simulink model "apilot3"  (Simulink 2.09)
settings: Solver=ode45  StartTime=0.0  StopTime=45  MaxStep=0.033  RelTol=1e-07  AbsTol=1e-05
values from neighbouring files (symbols this model uses):
  CD = 0    [apinit.m]    (also in vorinit.m)
  gamgs = -3*pi/180    (= -0.0523598775598)    [apinit.m]    (also in ilsinit.m = -3)
  HRW = 0    [apinit.m]    (also in ilsinit.m)
  Sgs = 625/abs(gamgs)    [apinit.m]    (also in ilsinit.m)
  Sloc = 1.4*xloc    (= 2800)    [apinit.m]    (also in ilsinit.m)
  xgs = 300    [apinit.m]    (also in ilsinit.m)
  xloc = 2000    [apinit.m]    (also in ilsinit.m)
  ymod1A = [1 1 1 0 0]'    [apmode.m]
  ymod1S = [1 1 1 0 0]'    [apmode.m]
  ymod2A = [1 1 0 0 1]'    [apmode.m]
  ymod2S = [1 1 0 0 1]'    [apmode.m]
  yrefA = [0 Dpsir]'    [apmode.m]
  yrefS = [0 0 DHdotr]'    [apmode.m]
undefined symbols (not defined in the file or in its folder): Aail, Aelv, AM, Arud, Bail, Belv, Brud, Cail, Celv, Crud, Dail, Delv, Drud, GM1, sfunyst, uaero0, uprop0, xdot0, xfix, xinco
libraries: navlib1 x5, wndlib2 x3, navlib2 x2, wndlib1 x1
(part 1 of 2)
settings Model: SaveTime=off  SaveOutput=off  ConsistencyChecking=off  RTWTemplateMakefile=grt_vc.tmf

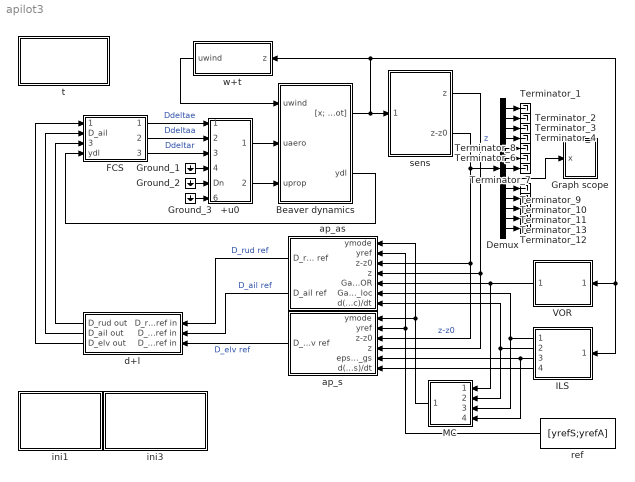
== system apilot3 ==
  +u0 : Subsystem
      mask Display: disp('Add\ninitial\ninputs')
  Beaver dynamics : Subsystem
  Demux : Demux  Outputs=13
  FCS : Subsystem
      mask Display: disp('Actuator &\ncable dy-\nnamics')
  Graph scope : Subsystem  mask(Storage scope.){npts=100, color='g-'}
      mask prompts: npts "Initial Time Range:"; color "Initial y-min:"
      mask help:
      | Storage scope using MATLAB graph window.
      | Enter plotting ranges and line type.
      mask init:
      | close all; ax = [0, @1, @2, @3];
      mask Help: Uses MATLAB's graph window.\nUse only one block per system.\nLine type must be in quotes.\nSee the M-file sfunyst.m.
      mask Display: plot(0,0,100,100,[83,76,63,52,42,38,28,16,11,84,11,11,11,90,90,11],[75,58,47,54,72,80,84,74,65,65,65,90,40,40,90,90])
  Ground_1 : Ground
  Ground_2 : Ground
  Ground_3 : Ground
  ILS : Subsystem  Orientation=left
      mask Display: plot(0,0,100,100,[53,23,30,61,53],[45,60,64,49,45],[16,27,32,26],[48,40,43,47],[21,20,24,26,21],[44,55,56,47,44],[20,20,16],[50,50,48],[38,27,26,33],[52,46,48,55],[42,38,27],[50,47,46],[40,44,44,45,45,44,42],[48,44,42,42,44,44,50],[47,45,43],[55,58,58],[54,84,98,90,54],[36,21,56,58,36],[74,68],[34,29],[81,76],[43,38],[87,83],[49,45],[94,89],[57,52],[105,105],[0,0])
  MC : Subsystem  Orientation=left
      mask Display: disp('Mode\nCon-\ntroller')
  Terminator_{1..4,6..13} (12 alike) : Terminator
  VOR : Subsystem  Orientation=left
      mask Display: plot(0,0,100,100,[86,85,90,86,80,85,0],[16,80,20,16,20,80,62],[22,18,25,28,22,19],[36,32,29,33,36,45],[17,15,12,18,16,19],[37,37,34,32,44,46],[22,31,47,52,19,15,28,22],[36,44,39,44,55,50,45,38],[31,28],[44,45],[20,18,17],[31,30,32],[36,35,36,37,36,35,35,35,33,31,25],[41,38,33,32,30,30,32,33,37,35,34],[85,42],[80,50],[86,87,87,86,84,83,84,85],[83,81,78,76,76,79,82,83])
  ap_as : Subsystem  Orientation=left
      mask Display: disp('Asymmetrical\nautopilot\nmodes')
  ap_s : Subsystem  Orientation=left
      mask Display: disp('Symmetrical\nautopilot\nmodes')
  d+l : Subsystem  Orientation=left
      mask Display: disp('computational\ndelay & limiters')
  ini1 : Subsystem
      settings: OpenFcn=apinit
      mask Type: apinit
      mask Display: disp('1. Initialize\nsubsystems\n\nAPINIT')
  ini3 : Subsystem
      settings: OpenFcn=apmode
      mask Type: apmode
      mask Display: disp('2. Select mode &\nreference signals\n\nAPMODE')
  ref : Constant  Orientation=left  Value=[yrefS;yrefA]
      mask Display: disp('Reference\nsignals')
  sens : Subsystem
      mask Display: disp('Sensors\n\nsubtract\ninitial\nconditions')
  t : Subsystem
      settings: OpenFcn=fdchelp apilot
      mask Display: disp('Apilot3\nMarc Rauw\nJune 2000')
  w+t : Subsystem  Orientation=left
      mask Display: disp('wind &\nturbulence')
  wires:
  Demux/8 -> Graph scope/1(x)
  Demux/5 -> Terminator_8/1
  Demux/6 -> Terminator_6/1
  Demux/13 -> Terminator_12/1
  Demux/12 -> Terminator_13/1
  Demux/11 -> Terminator_11/1
  Demux/10 -> Terminator_10/1
  Demux/9 -> Terminator_9/1
  Demux/4 -> Terminator_4/1
  Demux/7 -> Terminator_7/1
  Demux/3 -> Terminator_3/1
  Demux/2 -> Terminator_2/1
  Demux/1 -> Terminator_1/1
  Ground_3/1 -> +u0/6(Dpz)
  Ground_2/1 -> +u0/5(Dn)
  Ground_1/1 -> +u0/4(Ddeltaf)
  Beaver dynamics/1("[x; Hdot]") -> ILS/1("[x' ; Hdot]'"), VOR/1("[x' ; Hdot]'"), w+t/1(z), sens/1("[x; Hdot]")
  Beaver dynamics/2(ydl) -> FCS/4(ydl)
  VOR/1(Gamma_VOR) -> MC/1(Gamma_VOR), ap_as/5(Gamma_VOR)
  ap_s/1(D_elv ref) -> d+l/3(D_elv ref in)  "D_elv ref"
  d+l/3(D_elv out) -> FCS/1(D_elv)
  d+l/2(D_ail out) -> FCS/2(D_ail)
  d+l/1(D_rud out) -> FCS/3(D_rud)
  ref/1 -> ap_s/2(yref), ap_as/2(yref)
  MC/1(ymode) -> ap_s/1(ymode), ap_as/1(ymode)
  +u0/1(uaero) -> Beaver dynamics/2(uaero)
  sens/1(z) -> ap_as/4(z), ap_s/4(z)  "z"
  +u0/2(uprop) -> Beaver dynamics/3(uprop)
  FCS/1(Ddeltae) -> +u0/1(Ddeltae)  "Ddeltae"
  FCS/2(Ddeltaa) -> +u0/2(Ddeltaa)  "Ddeltaa"
  FCS/3(Ddeltar) -> +u0/3(Ddeltar)  "Ddeltar"
  ap_as/1(D_rud ref) -> d+l/1(D_rud ref in)  "D_rud ref"
  ap_as/2(D_ail ref) -> d+l/2(D_ail ref in)  "D_ail ref"
  w+t/1(uwind) -> Beaver dynamics/1(uwind)
  sens/2(z-z0) -> ap_s/3(z-z0), ap_as/3(z-z0), Demux/1  "z-z0"
  ILS/1(Gamma_loc) -> MC/3(Gamma_loc), ap_as/6(Gamma_loc)
  ILS/2(d(Gamma_loc)/dt) -> ap_as/7(d(Gamma_loc)/dt), MC/2(d(Gamma_loc)/dt)
  ILS/4(d(epsilon_gs)/dt) -> ap_s/6(d(epsilon_gs)/dt)
  ILS/3(epsilon_gs) -> ap_s/5(epsilon_gs), MC/4(epsilon_gs)

== system apilot3/+u0 ==
  note: AERODYNAMIC INPUTS:
  note: ENGINE INPUTS:
  note: Add initial inputs
  Ddeltae : Inport  Port=1  PortWidth=-1  SampleTime=-1
  Ddeltaa : Inport  Port=2  PortWidth=-1  SampleTime=-1
  Ddeltar : Inport  Port=3  PortWidth=-1  SampleTime=-1
  Ddeltaf : Inport  Port=4  PortWidth=-1  SampleTime=-1
  Dn : Inport  Port=5  PortWidth=-1  SampleTime=-1
  Dpz : Inport  Port=6  PortWidth=-1  SampleTime=-1
  Initial inputs for aeromod : Constant  Value=uaero0
  Initial inputs for engmod : Constant  Value=uprop0
  Mux1 : Mux  Inputs=4
  Mux2 : Mux  Inputs=2
  Sum : Sum  Inputs=++
  Sum1 : Sum  Inputs=++
  uaero : Outport  Port=1  InitialOutput=0
  uprop : Outport  Port=2  InitialOutput=0
  wires:
  Mux1/1 -> Sum1/2
  Sum1/1 -> uaero/1
  Initial inputs for aeromod/1 -> Sum1/1
  Ddeltaf/1 -> Mux1/4
  Ddeltar/1 -> Mux1/3
  Ddeltae/1 -> Mux1/1
  Ddeltaa/1 -> Mux1/2
  Sum/1 -> uprop/1
  Mux2/1 -> Sum/1
  Initial inputs for engmod/1 -> Sum/2
  Dn/1 -> Mux2/1
  Dpz/1 -> Mux2/2

== system apilot3/Beaver dynamics ==
  note: Beaver dynamics
      | and output equations
  uwind : Inport  Port=1  PortWidth=6  SampleTime=-1
  uaero : Inport  Port=2  PortWidth=4  SampleTime=-1
  uprop : Inport  Port=3  PortWidth=2  SampleTime=-1
  0 : Subsystem
      settings: OpenFcn=fdchelp level1
      mask Display: disp('Subsystem equivalent of\nthe S-function BEAVER\nM.O. Rauw, October 1997')
  AC : Subsystem
  Clock : Clock
  Demux1 : Demux  Outputs=[11 1]
  Mux : Mux  Inputs=[12 1]
  Mux_in : Mux  Orientation=up  Inputs=[4 2 6]
      settings: OpenFcn=fdchelp inputs
      mask Display: disp('Mux\nclick\n2x for\ninfo!')
  Mux_out : Mux  Orientation=up  Inputs=[12 12 3 3 3 4 2 6 6 6 6 6 3 3 5 3 3 3]
      settings: OpenFcn=fdchelp outputs
      mask Display: disp('Mux\n\nDouble-click for info!')
  Terminator_1 : Terminator
  To Workspace : ToWorkspace  VariableName=Out  SampleTime=0
      settings: Orientation=up  Buffer=5000
  "To Workspace " : ToWorkspace  VariableName=In  SampleTime=0
      settings: Orientation=up  Buffer=5000
  "To Workspace  " : ToWorkspace  VariableName=time  SampleTime=0
      settings: Buffer=5000
  "[x; Hdot]" : Outport  Port=1  InitialOutput=0
  ydl : Outport  Port=2  InitialOutput=0
  wires:
  AC/7(ypow) -> Mux_out/7
  Mux_in/1 -> "To Workspace "/1
  Mux_out/1 -> To Workspace/1
  Clock/1 -> "To Workspace  "/1
  AC/2(xdot) -> Mux_out/2, Demux1/1  "xdot"
  AC/15(yatm) -> Mux_out/15
  AC/14(Fwind) -> Mux_out/14
  AC/13(Fgrav) -> Mux_out/13
  AC/12(FMprop) -> Mux_out/12
  AC/11(FMaero) -> Mux_out/11
  AC/10(Cprop) -> Mux_out/10
  AC/9(Caero) -> Mux_out/9
  AC/8(yacc) -> Mux_out/8
  AC/6(yfp) -> Mux_out/6
  AC/5(ydl) -> ydl/1, Mux_out/5
  AC/16(yad1) -> Mux_out/16
  AC/3(ybvel) -> Mux_out/3
  AC/1(x) -> Mux/1, Mux_out/1  "x"
  AC/4(yuvw) -> Mux_out/4
  AC/17(yad2) -> Mux_out/17
  AC/18(yad3) -> Mux_out/18
  uwind/1 -> AC/3(" uwind"), Mux_in/3
  uprop/1 -> AC/2(uprop), Mux_in/2
  uaero/1 -> AC/1(uaero), Mux_in/1
  Demux1/1 -> Terminator_1/1
  Demux1/2 -> Mux/2  "Hdot"
  Mux/1 -> "[x; Hdot]"/1

== system apilot3/FCS ==
  note: Actuators
      | + cables:
  D_elv : Inport  Port=1  PortWidth=-1  SampleTime=-1
  D_ail : Inport  Port=2  PortWidth=-1  SampleTime=-1
  D_rud : Inport  Port=3  PortWidth=-1  SampleTime=-1
  ydl : Inport  Port=4  PortWidth=-1  SampleTime=-1
  Demux1 : Demux  Outputs=3
  Mux1 : Mux  Inputs=2
  Mux2 : Mux  Inputs=2
  Mux3 : Mux  Inputs=2
  ailerons : StateSpace  A=Aail  B=Bail  C=Cail*2  D=Dail  X0=0
  elevator : StateSpace  A=Aelv  B=Belv  C=Celv  D=Delv  X0=0
  rudder : StateSpace  A=Arud  B=Brud  C=Crud  D=Drud  X0=0
  t : Subsystem
      settings: OpenFcn=fdchelp actuatr
      mask Display: disp('Actuator & cable dynamics\nMarc Rauw, October 1997')
  Ddeltae : Outport  Port=1  InitialOutput=0
  Ddeltaa : Outport  Port=2  InitialOutput=0
  Ddeltar : Outport  Port=3  InitialOutput=0
  wires:
  D_rud/1 -> Mux3/1
  D_ail/1 -> Mux2/1
  D_elv/1 -> Mux1/1
  rudder/1 -> Ddeltar/1
  ydl/1 -> Demux1/1
  ailerons/1 -> Ddeltaa/1
  elevator/1 -> Ddeltae/1
  Mux3/1 -> rudder/1
  Mux2/1 -> ailerons/1
  Mux1/1 -> elevator/1
  Demux1/3 -> Mux3/2
  Demux1/1 -> Mux2/2
  Demux1/2 -> Mux1/2

== system apilot3/Graph scope ==
  x : Inport  Port=1  PortWidth=-1  SampleTime=-1
  "S-function M-file which plots lines " : S-Function  LoadFcn=sfunyst([],[],[],'LoadBlock')  FunctionName=sfunyst  Parameters=ax, color, npts
      settings: CopyFcn=sfunyst([],[],[],'CopyBlock')  DeleteFcn=sfunyst([],[],[],'DeleteBlock')
  wires:
  x/1 -> "S-function M-file which plots lines "/1

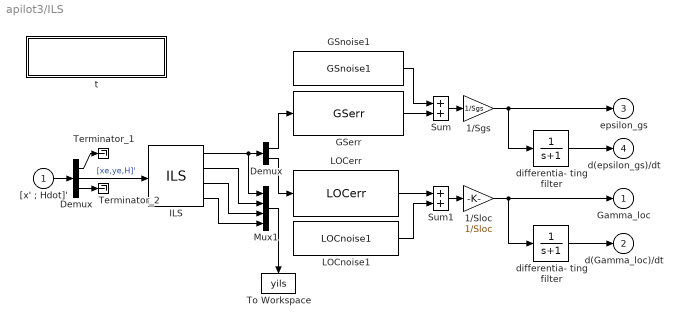
== system apilot3/ILS ==
  "[x' ; Hdot]'" : Inport  Port=1  PortWidth=-1  SampleTime=-1
  1/Sgs : Gain  Gain=1/Sgs
  1/Sloc : Gain  Gain=1/Sloc
  Demux : Demux  Outputs=2
  "Demux " : Demux  Outputs=[9 3 1]
  GSerr : navlib1/GSerr  cat=2  MaskParam2=100  MaskParam3=100  MaskParam4=-3
  GSnoise1 : navlib1/GSnoise1  Lgs=85  sigma_gs=15  V=40
  ILS : navlib1/ILS  RWpos=[20000,-100,0]  MaskParam1=0  MaskParam3=2200  MaskParam4=300  MaskParam5=100  MaskParam6=3
  LOCerr : navlib1/LOCerr  cat=2  xloc=2200  MaskParam2=100  MaskParam3=100
  LOCnoise1 : navlib1/LOCnoise1  Lloc=130  sigma_loc=15  V=40
  Mux1 : Mux  Inputs=[2 2 6 2]
  Sum : Sum  Inputs=++
  Sum1 : Sum  Inputs=++
  Terminator_1 : Terminator
  Terminator_2 : Terminator
  To Workspace : ToWorkspace  VariableName=yils  SampleTime=0
      settings: Orientation=down  Buffer=5000
  differentia- ting filter : TransferFcn  Numerator=[1]  Denominator=[1 1]
  "differentia- ting filter " : TransferFcn  Numerator=[1]  Denominator=[1 1]
  t : Subsystem
      mask Display: disp('ILS signals\nMarc Rauw, January 1998')
  Gamma_loc : Outport  Port=1  InitialOutput=0
  d(Gamma_loc)/dt : Outport  Port=2  InitialOutput=0
  epsilon_gs : Outport  Port=3  InitialOutput=0
  d(epsilon_gs)/dt : Outport  Port=4  InitialOutput=0
  wires:
  1/Sgs/1 -> epsilon_gs/1, "differentia- ting filter "/1
  "differentia- ting filter "/1 -> d(epsilon_gs)/dt/1
  1/Sloc/1 -> Gamma_loc/1, differentia- ting filter/1
  differentia- ting filter/1 -> d(Gamma_loc)/dt/1
  Mux1/1 -> To Workspace/1
  Demux/1 -> GSerr/1
  Demux/2 -> LOCerr/1
  GSerr/1 -> Sum/2
  LOCnoise1/1 -> Sum1/2
  Sum/1 -> 1/Sgs/1
  Sum1/1 -> 1/Sloc/1
  ILS/4 -> Mux1/4
  ILS/1 -> Demux/1, Mux1/1
  ILS/3 -> Mux1/3
  GSnoise1/1 -> Sum/1
  ILS/2 -> Mux1/2
  LOCerr/1 -> Sum1/1
  "Demux "/3 -> Terminator_2/1
  "Demux "/1 -> Terminator_1/1
  "Demux "/2 -> ILS/1  "[xe,ye,H]'"
  "[x' ; Hdot]'"/1 -> "Demux "/1

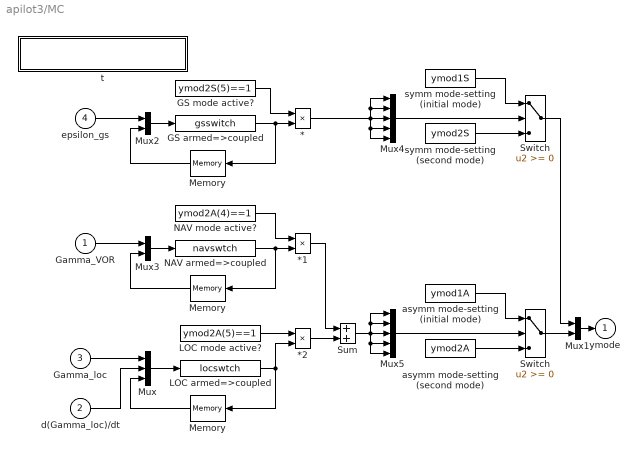
== system apilot3/MC ==
  Gamma_VOR : Inport  Port=1  PortWidth=-1  SampleTime=-1
  d(Gamma_loc)/dt : Inport  Port=2  PortWidth=-1  SampleTime=-1
  Gamma_loc : Inport  Port=3  PortWidth=-1  SampleTime=-1
  epsilon_gs : Inport  Port=4  PortWidth=-1  SampleTime=-1
  " Memory" : Memory  Orientation=left  X0=0  InheritSampleTime=off
  * : Product  Inputs=2
  *1 : Product  Inputs=2
  *2 : Product  Inputs=2
  GS armed=>coupled : MATLABFcn  MATLABFcn=gsswitch  OutputWidth=1
      mask Display: disp('gsswitch.m')
  GS mode active? : Constant  Value=ymod2S(5)==1
  LOC armed=>coupled : MATLABFcn  MATLABFcn=locswtch  OutputWidth=1
      mask Display: disp('locswtch.m')
  LOC mode active? : Constant  Value=ymod2A(5)==1
  Memory : Memory  Orientation=left  X0=1  InheritSampleTime=off
  "Memory " : Memory  Orientation=left  X0=0  InheritSampleTime=off
  Mux : Mux  Inputs=3
  Mux1 : Mux  Inputs=[5 5]
  Mux2 : Mux  Inputs=2
  Mux3 : Mux  Inputs=2
  Mux4 : Mux  Inputs=5
  Mux5 : Mux  Inputs=5
  NAV armed=>coupled : MATLABFcn  MATLABFcn=navswtch  OutputWidth=1
      mask Display: disp('navswtch.m')
  NAV mode active? : Constant  Value=ymod2A(4)==1
  Sum : Sum  Inputs=++
  Switch : Switch  Threshold=0
  "Switch " : Switch  Threshold=0
  asymm mode-setting (initial mode) : Constant  Value=ymod1A
  asymm mode-setting (second mode) : Constant  Value=ymod2A
  symm mode-setting (initial mode) : Constant  Value=ymod1S
  symm mode-setting (second mode) : Constant  Value=ymod2S
  t : Subsystem
      settings: OpenFcn=fdchelp modectrl
      mask Display: disp('Mode-controller\nM.O. Rauw, October 1997')
  ymode : Outport  Port=1  InitialOutput=0
  wires:
  asymm mode-setting (initial mode)/1 -> "Switch "/1
  symm mode-setting (initial mode)/1 -> Switch/1
  *1/1 -> Sum/1
  Sum/1 -> Mux5/2, Mux5/1, Mux5/4, Mux5/5, Mux5/3
  Switch/1 -> Mux1/1
  symm mode-setting (second mode)/1 -> Switch/3
  " Memory"/1 -> Mux/3
  "Memory "/1 -> Mux3/2
  Memory/1 -> Mux2/2
  */1 -> Mux4/4, Mux4/5, Mux4/2, Mux4/1, Mux4/3
  LOC armed=>coupled/1 -> " Memory"/1, *2/2
  asymm mode-setting (second mode)/1 -> "Switch "/3
  *2/1 -> Sum/2
  LOC mode active?/1 -> *2/1
  NAV mode active?/1 -> *1/1
  NAV armed=>coupled/1 -> *1/2, "Memory "/1
  GS mode active?/1 -> */1
  Mux1/1 -> ymode/1
  "Switch "/1 -> Mux1/2
  GS armed=>coupled/1 -> */2, Memory/1
  Mux5/1 -> "Switch "/2
  Mux4/1 -> Switch/2
  d(Gamma_loc)/dt/1 -> Mux/2
  Gamma_VOR/1 -> Mux3/1
  Mux3/1 -> NAV armed=>coupled/1
  epsilon_gs/1 -> Mux2/1
  Mux2/1 -> GS armed=>coupled/1
  Gamma_loc/1 -> Mux/1
  Mux/1 -> LOC armed=>coupled/1

== system apilot3/VOR ==
  "[x' ; Hdot]'" : Inport  Port=1  PortWidth=-1  SampleTime=-1
  Demux : Demux  Outputs=[6 1 2 3 1]
  Mux1 : Mux  Inputs=[1 1 2 1]
  Terminator_1 : Terminator
  Terminator_2 : Terminator
  Terminator_3 : Terminator
  To Workspace : ToWorkspace  VariableName=yvor  SampleTime=0
      settings: Buffer=5000
  VOR : navlib2/VOR  xVOR=xVOR  yVOR=yVOR  HVOR=HVOR  MaskParam4=CD
  VORERR : navlib2/VORERR  MaskParam1=5
  t : Subsystem
      mask Display: disp('VOR signals\nMarc Rauw, January 1998')
  Gamma_VOR : Outport  Port=1  InitialOutput=0
  wires:
  VOR/1 -> VORERR/1
  Mux1/1 -> To Workspace/1
  VOR/2 -> Mux1/2
  VOR/3 -> Mux1/3
  VOR/4 -> Mux1/4
  VORERR/1 -> Gamma_VOR/1, Mux1/1
  "[x' ; Hdot]'"/1 -> Demux/1
  Demux/5 -> Terminator_3/1
  Demux/3 -> Terminator_2/1
  Demux/1 -> Terminator_1/1
  Demux/4 -> VOR/1  "[xe,ye,H]'"
  Demux/2 -> VOR/2  "psi"

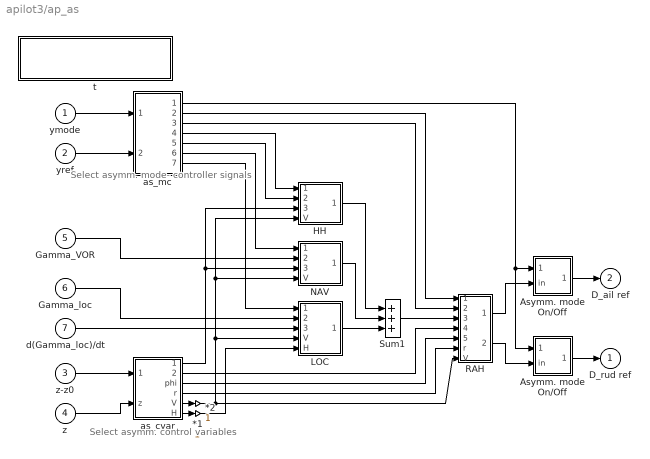
== system apilot3/ap_as ==
  note: Select asymm.
      | control variables
  note: Select asymm. mode-
      | controller signals
  ymode : Inport  Port=1  PortWidth=-1  SampleTime=-1
  yref : Inport  Port=2  PortWidth=-1  SampleTime=-1
  z-z0 : Inport  Port=3  PortWidth=-1  SampleTime=-1
  z : Inport  Port=4  PortWidth=-1  SampleTime=-1
  Gamma_VOR : Inport  Port=5  PortWidth=-1  SampleTime=-1
  Gamma_loc : Inport  Port=6  PortWidth=-1  SampleTime=-1
  d(Gamma_loc)/dt : Inport  Port=7  PortWidth=-1  SampleTime=-1
  *1 : Gain  Gain=1
  *2 : Gain  Gain=1
  Asymm. mode On/Off : Subsystem
      mask Type: On/off switch
      mask Description:
      | If input(1) = 1
      |      output = input(2)
      |  else if input(1) = 0
      |      output = 0
      mask Help: On/off switch.
      mask Display: plot(0,0,100,100,[31,31,32,34,34,32,31,31,0],[50,48,47,48,51,53,51,50,50],[100,75,51],[50,50,97]);disp('?')
  "Asymm. mode On/Off " : Subsystem
      mask Type: On/off switch
      mask Description:
      | If input(1) = 1
      |      output = input(2)
      |  else if input(1) = 0
      |      output = 0
      mask Help: On/off switch.
      mask Display: plot(0,0,100,100,[31,31,32,34,34,32,31,31,0],[50,48,47,48,51,53,51,50,50],[100,75,51],[50,50,97]);disp('?')
  HH : Subsystem
  LOC : Subsystem
  NAV : Subsystem
  RAH : Subsystem
  Sum1 : Sum  Inputs=+++
  as_cvar : Subsystem
  as_mc : Subsystem
  t : Subsystem
      settings: OpenFcn=fdchelp ap_asymm
      mask Display: disp('Asymm. autopilot modes\nMarc Rauw, October 1997')
  D_rud ref : Outport  Port=1  InitialOutput=0
  D_ail ref : Outport  Port=2  InitialOutput=0
  wires:
  as_mc/1(asymm. mode?) -> Asymm. mode On/Off/1(crit), "Asymm. mode On/Off "/1(crit)
  HH/1(Dphir (HH)) -> Sum1/1
  RAH/2(D_rud ref) -> Asymm. mode On/Off/2(in)
  RAH/1(D_ail ref) -> "Asymm. mode On/Off "/2(in)
  as_cvar/1(psi-psi0) -> NAV/3(psi-psi0), HH/3(psi-psi0)
  z-z0/1 -> as_cvar/1(z-z0)
  Asymm. mode On/Off/1(out) -> D_rud ref/1
  "Asymm. mode On/Off "/1(out) -> D_ail ref/1
  yref/1 -> as_mc/2(yref)
  ymode/1 -> as_mc/1(ymode)
  NAV/1(Dphir (NAV)) -> Sum1/2
  LOC/1(Dphir (LOC)) -> Sum1/3
  as_cvar/5(V) -> *1/1
  as_cvar/4(r) -> RAH/6(r)
  as_cvar/3(phi) -> RAH/5(phi)
  as_cvar/2(phi-phi0) -> RAH/4(phi-phi0)
  as_mc/2(asymm. out. loop?) -> RAH/1(Asymm out. loop?)
  as_mc/3(Dphir (RAH)) -> RAH/2(Dphir (RAH))
  as_mc/4(HH?) -> HH/1(HH?)
  as_mc/6(NAV?) -> NAV/1(NAV?)
  as_mc/7(LOC coupled?) -> LOC/1(LOC coupled?)
  as_cvar/6(H) -> *2/1
  *1/1 -> NAV/4(V), HH/4(V), LOC/4(V), RAH/7(V)
  *2/1 -> LOC/5(H)
  Sum1/1 -> RAH/3(Dphir (out. loop))
  as_mc/5(Dpsir (HH)) -> HH/2(Dpsir (HH))
  Gamma_VOR/1 -> NAV/2(Gamma_VOR)
  Gamma_loc/1 -> LOC/2(Gamma_loc)
  d(Gamma_loc)/dt/1 -> LOC/3(d(Gamma_loc)/dt)
  z/1 -> as_cvar/2(z)

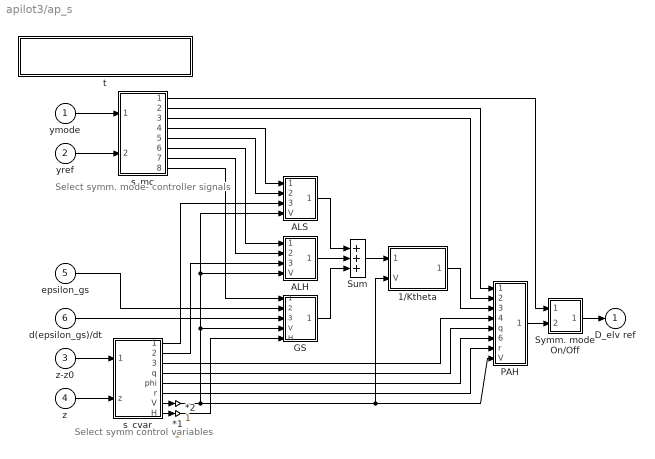
== system apilot3/ap_s ==
  note: Select symm
      | control variables
  note: Select symm. mode-
      | controller signals
  ymode : Inport  Port=1  PortWidth=-1  SampleTime=-1
  yref : Inport  Port=2  PortWidth=-1  SampleTime=-1
  z-z0 : Inport  Port=3  PortWidth=-1  SampleTime=-1
  z : Inport  Port=4  PortWidth=-1  SampleTime=-1
  epsilon_gs : Inport  Port=5  PortWidth=-1  SampleTime=-1
  d(epsilon_gs)/dt : Inport  Port=6  PortWidth=-1  SampleTime=-1
  *1 : Gain  Gain=1
  *2 : Gain  Gain=1
  1/Ktheta : Subsystem
      mask Display: plot(0,0,100,100,[0,100,0],[0,50,100]);disp('K(u1)      ')
  ALH : Subsystem
  ALS : Subsystem
  GS : Subsystem
  PAH : Subsystem
  Sum : Sum  Inputs=+++
  Symm. mode On/Off : Subsystem
      mask Type: On/off switch
      mask Description:
      | If input(1) = 1
      |      output = input(2)
      |  else if input(1) = 0
      |      output = 0
      mask Help: On/off switch. \nIf input(1) = 1, the output equals input(1). \nIf input(1) = 0, the output is zero.
      mask Display: plot(0,0,100,100,[31,31,32,34,34,32,31,31,0],[50,48,47,48,51,53,51,50,50],[100,75,51],[50,50,97]);disp('?')
  s_cvar : Subsystem
  s_mc : Subsystem
  t : Subsystem
      settings: OpenFcn=fdchelp ap_symm
      mask Display: disp('Symm. autopilot modes\nMarc Rauw, October 1997')
  D_elv ref : Outport  Port=1  InitialOutput=0
  wires:
  s_mc/8(GS coupled?) -> GS/1(GS coupled?)
  *2/1 -> GS/5(H)
  s_cvar/8(H) -> *2/1
  yref/1 -> s_mc/2(yref)
  ymode/1 -> s_mc/1(ymode)
  s_mc/7(DHr (ALH)) -> ALH/2(DHr (ALH))
  s_mc/6(ALH?) -> ALH/1(ALH?)
  s_mc/5(DHdot r (ALS)) -> ALS/2(DHdot r (ALS))
  s_mc/4(ALS?) -> ALS/1(ALS?)
  s_mc/3(Dthetar (PAH)) -> PAH/2(Dthetar (PAH/GA))
  s_mc/2(symm. outer loop?) -> PAH/1(Symm out. loop?)
  z/1 -> s_cvar/2(z)
  z-z0/1 -> s_cvar/1(z-z0)
  s_cvar/7(V) -> *1/1
  s_cvar/6(r) -> PAH/7(r)
  s_cvar/5(phi) -> PAH/6(phi)
  s_cvar/4(q) -> PAH/5(q)
  s_cvar/3(theta-theta0) -> PAH/4(theta-theta0)
  s_cvar/2(H-H0) -> ALH/3(H-H0)
  s_cvar/1(Hdot-Hdot0) -> ALS/3(Hdot-Hdot0)
  ALH/1(Dthetar (ALH)) -> Sum/2
  ALS/1(Dthetar (ALS)) -> Sum/1
  PAH/1(D_elv ref) -> Symm. mode On/Off/2(in)
  Symm. mode On/Off/1(out) -> D_elv ref/1
  s_mc/1(symm mode?) -> Symm. mode On/Off/1(crit)
  GS/1(Dthetar (GS)) -> Sum/3
  Sum/1 -> 1/Ktheta/1(input u)
  1/Ktheta/1(y = K*u) -> PAH/3(Dthetar (out. loop))
  *1/1 -> GS/4(V), ALH/4(V), ALS/4(V), 1/Ktheta/2(V), PAH/8(V)
  d(epsilon_gs)/dt/1 -> GS/3(d(epsilon_gs)/dt)
  epsilon_gs/1 -> GS/2(epsilon_gs)

== system apilot3/d+l ==
  D_rud ref in : Inport  Port=1  PortWidth=-1  SampleTime=-1
  D_ail ref in : Inport  Port=2  PortWidth=-1  SampleTime=-1
  D_elv ref in : Inport  Port=3  PortWidth=-1  SampleTime=-1
  " +/- 10 V " : Saturate  UpperLimit=10 * (pi/180)  LowerLimit=-10 * (pi/180)
  " delay" : TransportDelay  DelayTime=0.03  InitialInput=0  BufferSize=1024
  +/- 10 V : Saturate  UpperLimit=10 * (pi/180)  LowerLimit=-10 * (pi/180)
  "+/- 10 V " : Saturate  UpperLimit=10 * (pi/180)  LowerLimit=-10 * (pi/180)
  delay : TransportDelay  DelayTime=0.03  InitialInput=0  BufferSize=1024
  "delay " : TransportDelay  DelayTime=0.03  InitialInput=0  BufferSize=1024
  t : Subsystem
      settings: OpenFcn=fdchelp delaylim
      mask Display: disp('Computational delay and\ninput limiters (+- 10 Volt)\nMarc Rauw, October 1997')
  D_rud out : Outport  Port=1  InitialOutput=0
  D_ail out : Outport  Port=2  InitialOutput=0
  D_elv out : Outport  Port=3  InitialOutput=0
  wires:
  "delay "/1 -> "+/- 10 V "/1
  " delay"/1 -> " +/- 10 V "/1
  +/- 10 V/1 -> D_rud out/1
  "+/- 10 V "/1 -> D_ail out/1
  D_ail ref in/1 -> "delay "/1
  " +/- 10 V "/1 -> D_elv out/1
  D_elv ref in/1 -> " delay"/1
  delay/1 -> +/- 10 V/1
  D_rud ref in/1 -> delay/1

== system apilot3/ini1 ==

== system apilot3/ini3 ==

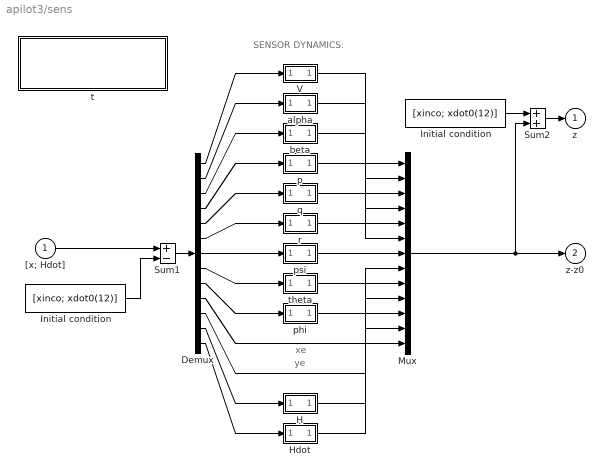
== system apilot3/sens ==
  note: SENSOR DYNAMICS:
  note: xe
  note: ye
  "[x; Hdot]" : Inport  Port=1  PortWidth=-1  SampleTime=-1
  Demux : Demux  Outputs=13
  H : Subsystem
  Hdot : Subsystem
  Initial condition : Constant  Value=[xinco; xdot0(12)]
  "Initial condition " : Constant  Value=[xinco; xdot0(12)]
  Mux : Mux  Inputs=13
  Sum1 : Sum  Inputs=+-
  Sum2 : Sum  Inputs=++
  V : Subsystem
  alpha : Subsystem
  beta : Subsystem
  p : Subsystem
  phi : Subsystem
  psi : Subsystem
  q : Subsystem
  r : Subsystem
  t : Subsystem
      settings: OpenFcn=fdchelp sensors
      mask Display: disp('Include sensormodels\nhere (no VOR/ILS)!\nMarc Rauw, October 1997')
  theta : Subsystem
  z : Outport  Port=1  InitialOutput=0
  z-z0 : Outport  Port=2  InitialOutput=0
  wires:
  Sum1/1 -> Demux/1
  "[x; Hdot]"/1 -> Sum1/1
  Initial condition/1 -> Sum1/2
  Hdot/1(Hdot out) -> Mux/13
  H/1(H out) -> Mux/12
  V/1(V out) -> Mux/1
  alpha/1(alpha out) -> Mux/2
  beta/1(beta out) -> Mux/3
  p/1(p out) -> Mux/4
  q/1(q out) -> Mux/5
  r/1(r out) -> Mux/6
  psi/1(psi out) -> Mux/7
  theta/1(theta out) -> Mux/8
  phi/1(phi out) -> Mux/9
  Demux/13 -> Hdot/1(Hdot in)
  Demux/12 -> H/1(H in)
  Demux/11 -> Mux/11
  Demux/10 -> Mux/10
  Demux/9 -> phi/1(phi in)
  Demux/8 -> theta/1(theta in)
  Demux/7 -> psi/1(psi in)
  Demux/6 -> r/1(r in)
  Demux/5 -> q/1(q in)
  Demux/4 -> p/1(p in)
  Demux/3 -> beta/1(beta in)
  Demux/2 -> alpha/1(alpha in)
  Demux/1 -> V/1(V in)
  "Initial condition "/1 -> Sum2/1
  Sum2/1 -> z/1
  Mux/1 -> Sum2/2, z-z0/1

== system apilot3/t ==

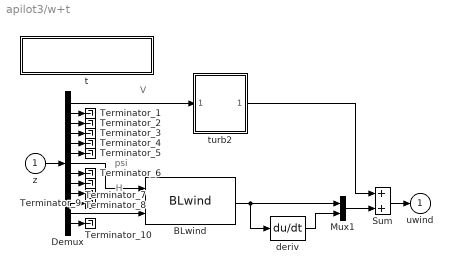
== system apilot3/w+t ==
  note: H
  note: psi
  note: V
  z : Inport  Port=1  PortWidth=-1  SampleTime=-1
  BLwind : wndlib1/BLwind
  Demux : Demux  Outputs=13
  Mux1 : Mux  Inputs=[3 3]
  Sum : Sum  Inputs=++
  Terminator_{1..10} (10 alike) : Terminator
  deriv : Derivative
  t : Subsystem
      mask Display: disp('Wind and turbulence\nMarc Rauw, January 1998')
  turb2 : Subsystem
  uwind : Outport  Port=1  InitialOutput=0
  wires:
  Demux/13 -> Terminator_10/1
  Demux/11 -> Terminator_9/1
  Demux/10 -> Terminator_8/1
  Demux/9 -> Terminator_7/1
  Demux/8 -> Terminator_6/1
  Demux/6 -> Terminator_5/1
  Demux/5 -> Terminator_4/1
  Demux/4 -> Terminator_3/1
  Demux/3 -> Terminator_2/1
  Demux/2 -> Terminator_1/1
  z/1 -> Demux/1
  Demux/7 -> BLwind/1
  Demux/12 -> BLwind/2
  BLwind/1 -> deriv/1, Mux1/1
  deriv/1 -> Mux1/2
  Sum/1 -> uwind/1
  Demux/1 -> turb2/1(V [m/s])
  turb2/1(uwind (due to turbulence)) -> Sum/1
  Mux1/1 -> Sum/2

== system apilot3/Beaver dynamics/0 ==

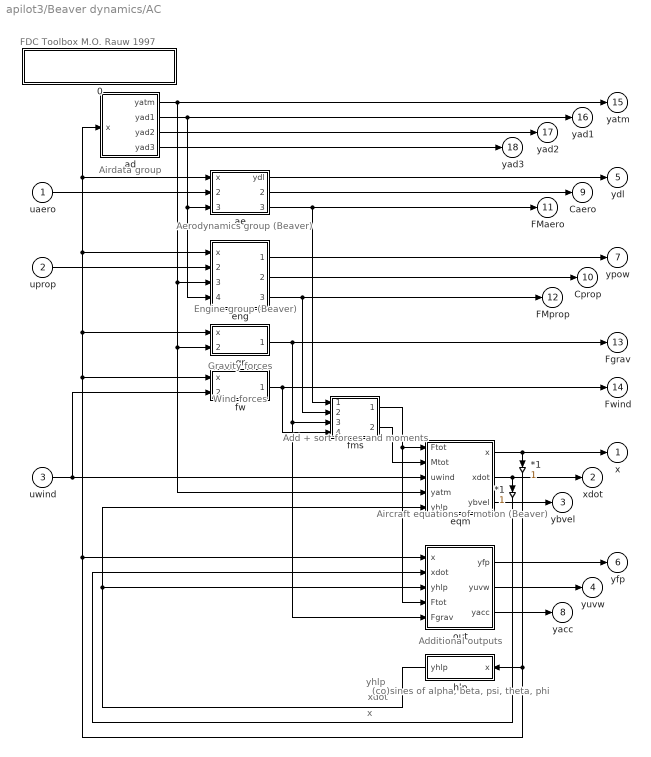
== system apilot3/Beaver dynamics/AC ==
  note: FDC Toolbox
      |  M.O. Rauw 1997
  note: xdot
  note: x
  note: yhlp
  note: Additional outputs
  note: Aircraft equations
      | of motion (Beaver)
  note: Wind forces
  note: Gravity forces
  note: Engine group (Beaver)
  note: Aerodynamics
      | group (Beaver)
  note: (co)sines of
      | alpha, beta,
      | psi, theta, phi
  note: Add + sort
      | forces and
      | moments
  note: Airdata group
  uaero : Inport  Port=1  PortWidth=-1  SampleTime=-1
  uprop : Inport  Port=2  PortWidth=-1  SampleTime=-1
  " uwind" : Inport  Port=3  PortWidth=-1  SampleTime=-1
  " *1" : Gain  Orientation=down  Gain=1
  *1 : Gain  Orientation=down  Gain=1
  0 : Subsystem
      settings: OpenFcn=fdchelp level2
      mask Display: disp('BEAVER, level 2 (main level)\nM.O. Rauw')
  ad : Subsystem
  ae : Subsystem
  eng : Subsystem
  eqm : Subsystem
  fms : Subsystem
      mask Type: FMsort
      mask Description: Forces and Moments sorting block
      mask Help: eval('fdchelp fmsort')
      mask Display: disp('FMsort')
  fw : Subsystem  mask(fwind){m=GM1(10)}
      mask prompts: m "Mass of the aircraft [kg]:"
      mask help: Forces due to non-steady atmosphere.
      mask Help: eval('fdchelp fwind')
      mask Display: disp('Fwind')
  gr : Subsystem  mask(Gravity){m=GM1(10)}
      mask prompts: m "Mass of the aircraft [kg]:"
      mask help: Gravity forces.
      mask Help: eval('fdchelp gravity')
      mask Display: disp('Gravity')
  hlp : Subsystem  Orientation=left
      mask Type: Hlpfcn
      mask Description: Help sines and cosines
      mask Help: eval('fdchelp hlpfcn')
      mask Display: disp('hlpfcn')
  out : Subsystem
  x : Outport  Port=1  InitialOutput=0
  xdot : Outport  Port=2  InitialOutput=0
  ybvel : Outport  Port=3  InitialOutput=0
  yuvw : Outport  Port=4  InitialOutput=0
  ydl : Outport  Port=5  InitialOutput=0
  yfp : Outport  Port=6  InitialOutput=0
  ypow : Outport  Port=7  InitialOutput=0
  yacc : Outport  Port=8  InitialOutput=0
  Caero : Outport  Port=9  InitialOutput=0
  Cprop : Outport  Port=10  InitialOutput=0
  FMaero : Outport  Port=11  InitialOutput=0
  FMprop : Outport  Port=12  InitialOutput=0
  Fgrav : Outport  Port=13  InitialOutput=0
  Fwind : Outport  Port=14  InitialOutput=0
  yatm : Outport  Port=15  InitialOutput=0
  yad1 : Outport  Port=16  InitialOutput=0
  yad2 : Outport  Port=17  InitialOutput=0
  yad3 : Outport  Port=18  InitialOutput=0
  wires:
  out/2(yuvw) -> yuvw/1
  uprop/1 -> eng/2(uprop)
  uaero/1 -> ae/2(uaero)
  ad/4(yad3) -> yad3/1
  ae/1(ydl) -> ydl/1
  ae/2(Caero) -> Caero/1
  eng/1(ypow) -> ypow/1
  eng/2(Cprop) -> Cprop/1
  eqm/3(ybvel) -> ybvel/1
  out/1(yfp) -> yfp/1
  ad/2(yad1) -> eng/4(yad1), ae/3(yad1), yad1/1
  ad/3(yad2) -> yad2/1
  ad/1(yatm) -> yatm/1, eng/3(yatm), eqm/4(yatm), gr/2(yatm)
  out/3(yacc) -> yacc/1
  fw/1(Fwind) -> Fwind/1, fms/4(Fwind)
  eng/3(FMprop) -> FMprop/1, fms/2(FMprop)
  ae/3(FMaero) -> FMaero/1, fms/1(FMaero)
  hlp/1(yhlp) -> eqm/5(yhlp), out/3(yhlp)
  " uwind"/1 -> eqm/3(uwind), fw/2(uwind)
  *1/1 -> out/2(xdot)
  gr/1(Fgrav) -> Fgrav/1, fms/3(Fgrav), out/5(Fgrav)
  " *1"/1 -> hlp/1(x), out/1(x), fw/1(x), gr/1(x), eng/1(x), ae/1(x), ad/1(x)
  eqm/2(xdot) -> xdot/1, *1/1
  eqm/1(x) -> x/1, " *1"/1
  fms/1(Ftot) -> out/4(Ftot), eqm/1(Ftot)
  fms/2(Mtot) -> eqm/2(Mtot)

== system apilot3/FCS/t ==

== system apilot3/ILS/t ==

== system apilot3/MC/t ==

== system apilot3/VOR/t ==

== system apilot3/ap_as/Asymm. mode On/Off ==
  crit : Inport  Port=1  PortWidth=-1  SampleTime=-1
  in : Inport  Port=2  PortWidth=-1  SampleTime=-1
  Sum : Sum  Inputs=+-
  Switch : Switch  Threshold=0
  const. : Constant  Value=0.5
  const.1 : Constant  Value=0
  out : Outport  Port=1  InitialOutput=0
  wires:
  crit/1 -> Sum/1
  const.1/1 -> Switch/3
  Sum/1 -> Switch/2
  Switch/1 -> out/1
  in/1 -> Switch/1
  const./1 -> Sum/2

== system apilot3/ap_as/Asymm. mode On/Off  ==
  crit : Inport  Port=1  PortWidth=-1  SampleTime=-1
  in : Inport  Port=2  PortWidth=-1  SampleTime=-1
  Sum : Sum  Inputs=+-
  Switch : Switch  Threshold=0
  const. : Constant  Value=0.5
  const.1 : Constant  Value=0
  out : Outport  Port=1  InitialOutput=0
  wires:
  const./1 -> Sum/2
  in/1 -> Switch/1
  Switch/1 -> out/1
  Sum/1 -> Switch/2
  const.1/1 -> Switch/3
  crit/1 -> Sum/1

== system apilot3/ap_as/HH ==
  note: Heading Hold / Heading Select mode
  HH? : Inport  Port=1  PortWidth=-1  SampleTime=-1
  Dpsir (HH) : Inport  Port=2  PortWidth=-1  SampleTime=-1
  psi-psi0 : Inport  Port=3  PortWidth=-1  SampleTime=-1
  V : Inport  Port=4  PortWidth=-1  SampleTime=-1
  Kpsi : Subsystem
      mask Display: plot(0,0,100,100,[0,100,0],[0,50,100]);disp('K(u1)      ')
  On/Off : Subsystem
      mask Type: On/off switch
      mask Description:
      | If input(1) = 1
      |      output = input(2)
      |  else if input(1) = 0
      |      output = 0
      mask Help: On/off switch.
      mask Display: plot(0,0,100,100,[31,31,32,34,34,32,31,31,0],[50,48,47,48,51,53,51,50,50],[100,75,51],[50,50,97]);disp('?')
  Sum : Sum  Inputs=+-
  Dphir (HH) : Outport  Port=1  InitialOutput=0
  wires:
  On/Off/1(out) -> Dphir (HH)/1
  Sum/1 -> Kpsi/2(input u)
  Kpsi/1(y = K*u) -> On/Off/2(in)
  psi-psi0/1 -> Sum/2
  Dpsir (HH)/1 -> Sum/1
  HH?/1 -> On/Off/1(crit)
  V/1 -> Kpsi/1(V)

== system apilot3/ap_as/LOC ==
  note: Localizer coupled mode
  LOC coupled? : Inport  Port=1  PortWidth=-1  SampleTime=-1
  Gamma_loc : Inport  Port=2  PortWidth=-1  SampleTime=-1
  d(Gamma_loc)/dt : Inport  Port=3  PortWidth=-1  SampleTime=-1
  V : Inport  Port=4  PortWidth=-1  SampleTime=-1
  H : Inport  Port=5  PortWidth=-1  SampleTime=-1
  KGam_LOC : Subsystem
      mask Display: plot(0,0,100,100,[0,100,0],[0,50,100]);disp('K(u1)       ')
  Kv : Gain  Gain=10
  On/Off : Subsystem
      mask Type: On/off switch
      mask Description:
      | If input(1) = 1
      |      output = input(2)
      |  else if input(1) = 0
      |      output = 0
      mask Help: On/off switch.
      mask Display: plot(0,0,100,100,[31,31,32,34,34,32,31,31,0],[50,48,47,48,51,53,51,50,50],[100,75,51],[50,50,97]);disp('?')
  Rloc approximation : Fcn  Expr=(u[1]-HRW)/sin(abs(gamgs*pi/180)) + xloc
  Sum : Sum  Inputs=++
  prod : Product  Inputs=2
  Dphir (LOC) : Outport  Port=1  InitialOutput=0
  wires:
  Rloc approximation/1 -> prod/2
  On/Off/1(out) -> Dphir (LOC)/1
  LOC coupled?/1 -> On/Off/1(crit)
  KGam_LOC/1(y = K*u) -> On/Off/2(in)
  prod/1 -> KGam_LOC/2(input u)
  H/1 -> Rloc approximation/1
  Sum/1 -> prod/1
  d(Gamma_loc)/dt/1 -> Kv/1
  Kv/1 -> Sum/2
  Gamma_loc/1 -> Sum/1
  V/1 -> KGam_LOC/1(V)

== system apilot3/ap_as/NAV ==
  note: VOR navigation mode
  NAV? : Inport  Port=1  PortWidth=-1  SampleTime=-1
  Gamma_VOR : Inport  Port=2  PortWidth=-1  SampleTime=-1
  psi-psi0 : Inport  Port=3  PortWidth=-1  SampleTime=-1
  V : Inport  Port=4  PortWidth=-1  SampleTime=-1
  Dpsir (NAV) : Constant  Value=CD-xinco(7)
  KGam_VOR : Subsystem
      mask Display: plot(0,0,100,100,[0,100,0],[0,50,100]);disp('K(u1)     ')
  Kpsi : Subsystem
      mask Display: plot(0,0,100,100,[0,100,0],[0,50,100]);disp('K(u1)      ')
  Low-pass filter : TransferFcn  Numerator=[1]  Denominator=[1 1]
  On/Off : Subsystem
      mask Type: On/off switch
      mask Description:
      | If input(1) = 1
      |      output = input(2)
      |  else if input(1) = 0
      |      output = 0
      mask Help: On/off switch.
      mask Display: plot(0,0,100,100,[31,31,32,34,34,32,31,31,0],[50,48,47,48,51,53,51,50,50],[100,75,51],[50,50,97]);disp('?')
  Sum : Sum  Inputs=++
  Sum1 : Sum  Inputs=+-
  Washout filter (includes forward loop below) : TransferFcn  Numerator=[15 0]  Denominator=[15 1]
  Dphir (NAV) : Outport  Port=1  InitialOutput=0
  wires:
  Dpsir (NAV)/1 -> Sum1/1
  Sum1/1 -> Kpsi/2(input u)
  Gamma_VOR/1 -> KGam_VOR/2(input u)
  KGam_VOR/1(y = K*u) -> Low-pass filter/1
  Low-pass filter/1 -> Sum/1
  Kpsi/1(y = K*u) -> Washout filter (includes forward loop below)/1
  Washout filter (includes forward loop below)/1 -> Sum/2
  Sum/1 -> On/Off/2(in)
  On/Off/1(out) -> Dphir (NAV)/1
  NAV?/1 -> On/Off/1(crit)
  psi-psi0/1 -> Sum1/2
  V/1 -> KGam_VOR/1(V), Kpsi/1(V)

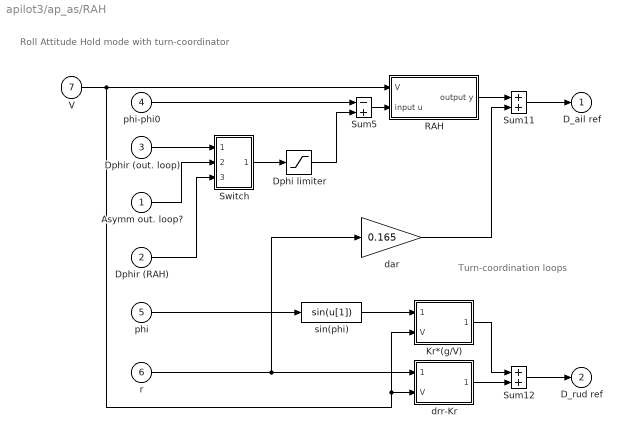
== system apilot3/ap_as/RAH ==
  note: Roll Attitude Hold mode
      | with turn-coordinator
  note: Turn-coordination loops
  Asymm out. loop? : Inport  Port=1  PortWidth=-1  SampleTime=-1
  Dphir (RAH) : Inport  Port=2  PortWidth=-1  SampleTime=-1
  Dphir (out. loop) : Inport  Port=3  PortWidth=-1  SampleTime=-1
  phi-phi0 : Inport  Port=4  PortWidth=-1  SampleTime=-1
  phi : Inport  Port=5  PortWidth=-1  SampleTime=-1
  r : Inport  Port=6  PortWidth=-1  SampleTime=-1
  V : Inport  Port=7  PortWidth=-1  SampleTime=-1
  Dphi limiter : Saturate  UpperLimit=30*pi/180  LowerLimit=-30*pi/180
  Kr*(g/V) : Subsystem
      mask Display: plot(0,0,100,100,[0,100,0],[0,50,100]);disp('K(u2)      ')
  RAH : Subsystem
      mask Display: disp('RAH (limited \n PI controller)')
  Sum11 : Sum  Inputs=++
  Sum12 : Sum  Inputs=++
  Sum5 : Sum  Inputs=-+
  Switch : Subsystem
      mask Display: plot(0,0,100,100,[100,70,40,0],[50,50,80,80],[40,0],[20,20],[29,29,0],[64,50,50],[29,29],[36,50],[40,40,41,40,39,40],[80,82,80,78,80,82],[40,40,41,40,39,40],[19,21,20,18,20,23])
  dar : Gain  Gain=0.165
  drr-Kr : Subsystem
      mask Display: plot(0,0,100,100,[0,100,0],[0,50,100]);disp('K(u2)      ')
  sin(phi) : Fcn  Expr=sin(u[1])
  D_ail ref : Outport  Port=1  InitialOutput=0
  D_rud ref : Outport  Port=2  InitialOutput=0
  wires:
  Dphir (RAH)/1 -> Switch/3(Dphir (RAH))
  Asymm out. loop?/1 -> Switch/2(Asymm.  out. loop?)
  Dphir (out. loop)/1 -> Switch/1(Dphir (out. loop))
  r/1 -> dar/1, drr-Kr/1(input u)
  Dphi limiter/1 -> Sum5/2
  Sum5/1 -> RAH/2(input u)
  dar/1 -> Sum11/2
  Kr*(g/V)/1(y = K*u) -> Sum12/1
  sin(phi)/1 -> Kr*(g/V)/1(input u)
  drr-Kr/1(y = K*u) -> Sum12/2
  Sum12/1 -> D_rud ref/1
  Sum11/1 -> D_ail ref/1
  RAH/1(output y) -> Sum11/1
  Switch/1(Dphir) -> Dphi limiter/1
  phi-phi0/1 -> Sum5/1
  phi/1 -> sin(phi)/1
  V/1 -> drr-Kr/2(V), Kr*(g/V)/2(V), RAH/1(V)

== system apilot3/ap_as/as_cvar ==
  note: True values of output
      | signals from AC model:
  note: Deviations from nominal
      | outputs from AC model:
  note: SELECT MEASURED ASYMM MOTION VARIABLES
  note: p
  z-z0 : Inport  Port=1  PortWidth=-1  SampleTime=-1
  z : Inport  Port=2  PortWidth=-1  SampleTime=-1
  Demux : Demux  Outputs=[6 1 1 1 4]
  Demux1 : Demux  Outputs=[1 2 1 1 1 2 1 2 1 1]
  Terminator_{1..9} (9 alike) : Terminator
  psi-psi0 : Outport  Port=1  InitialOutput=0
  phi-phi0 : Outport  Port=2  InitialOutput=0
  phi : Outport  Port=3  InitialOutput=0
  r : Outport  Port=4  InitialOutput=0
  V : Outport  Port=5  InitialOutput=0
  H : Outport  Port=6  InitialOutput=0
  wires:
  Demux1/1 -> V/1
  Demux1/10 -> Terminator_8/1
  Demux1/8 -> Terminator_7/1
  Demux1/6 -> Terminator_6/1
  Demux1/4 -> Terminator_5/1
  Demux1/2 -> Terminator_4/1
  Demux1/7 -> phi/1
  Demux1/5 -> r/1
  Demux1/3 -> Terminator_9/1
  z/1 -> Demux1/1
  Demux1/9 -> H/1
  Demux/5 -> Terminator_3/1
  Demux/3 -> Terminator_2/1
  Demux/1 -> Terminator_1/1
  Demux/4 -> phi-phi0/1
  Demux/2 -> psi-psi0/1
  z-z0/1 -> Demux/1

== system apilot3/ap_as/as_mc ==
  note: SELECT ASYMM REFERENCE SIGNALS
  note: SELECT ASYMM MODE (on/off flags denoted by '?')
  ymode : Inport  Port=1  PortWidth=-1  SampleTime=-1
  yref : Inport  Port=2  PortWidth=-1  SampleTime=-1
  Demux : Demux  Outputs=[5 1 1 1 1 1]
  Demux1 : Demux  Outputs=[3 1 1]
  Terminator_1 : Terminator
  Terminator_2 : Terminator
  asymm. mode? : Outport  Port=1  InitialOutput=0
  asymm. out. loop? : Outport  Port=2  InitialOutput=0
  Dphir (RAH) : Outport  Port=3  InitialOutput=0
  HH? : Outport  Port=4  InitialOutput=0
  Dpsir (HH) : Outport  Port=5  InitialOutput=0
  NAV? : Outport  Port=6  InitialOutput=0
  LOC coupled? : Outport  Port=7  InitialOutput=0
  wires:
  Demux1/1 -> Terminator_2/1
  Demux/1 -> Terminator_1/1
  Demux/6 -> LOC coupled?/1
  Demux/5 -> NAV?/1
  Demux/4 -> HH?/1
  Demux/3 -> asymm. out. loop?/1
  Demux/2 -> asymm. mode?/1
  ymode/1 -> Demux/1
  Demux1/3 -> Dpsir (HH)/1
  Demux1/2 -> Dphir (RAH)/1
  yref/1 -> Demux1/1

== system apilot3/ap_as/t ==

== system apilot3/ap_s/1/Ktheta ==
  input u : Inport  Port=1  PortWidth=-1  SampleTime=-1
  V : Inport  Port=2  PortWidth=-1  SampleTime=-1
  1/Ktheta : Fcn  Expr=1/(-1.375*10^(-3)*u[1]^2 + 0.1575*u[1] - 4.8031)
  Product : Product  Inputs=2
  y = K*u : Outport  Port=1  InitialOutput=0
  wires:
  1/Ktheta/1 -> Product/1
  input u/1 -> Product/2
  Product/1 -> y = K*u/1
  V/1 -> 1/Ktheta/1

== system apilot3/ap_s/ALH ==
  note: Altitude Hold mode
  ALH? : Inport  Port=1  PortWidth=-1  SampleTime=-1
  DHr (ALH) : Inport  Port=2  PortWidth=-1  SampleTime=-1
  H-H0 : Inport  Port=3  PortWidth=-1  SampleTime=-1
  V : Inport  Port=4  PortWidth=-1  SampleTime=-1
  KH : Subsystem
      mask Display: plot(0,0,100,100,[0,100,0],[0,50,100]);disp('K(u1)      ')
  On/Off : Subsystem
      mask Type: On/off switch
      mask Description:
      | If input(1) = 1
      |      output = input(2)
      |  else if input(1) = 0
      |      output = 0
      mask Help: On/off switch.
      mask Display: plot(0,0,100,100,[31,31,32,34,34,32,31,31,0],[50,48,47,48,51,53,51,50,50],[100,75,51],[50,50,97]);disp('?')
  Sum : Sum  Inputs=+-
  Dthetar (ALH) : Outport  Port=1  InitialOutput=0
  wires:
  H-H0/1 -> Sum/2
  On/Off/1(out) -> Dthetar (ALH)/1
  DHr (ALH)/1 -> Sum/1
  ALH?/1 -> On/Off/1(crit)
  KH/1(y = K*u) -> On/Off/2(in)
  Sum/1 -> KH/2(input u)
  V/1 -> KH/1(V)

== system apilot3/ap_s/ALS ==
  note: Altitude Select Mode
  ALS? : Inport  Port=1  PortWidth=-1  SampleTime=-1
  DHdot r (ALS) : Inport  Port=2  PortWidth=-1  SampleTime=-1
  Hdot-Hdot0 : Inport  Port=3  PortWidth=-1  SampleTime=-1
  V : Inport  Port=4  PortWidth=-1  SampleTime=-1
  KHdot : Subsystem
      mask Display: plot(0,0,100,100,[0,100,0],[0,50,100]);disp('K(u1)      ')
  On/Off : Subsystem
      mask Type: On/off switch
      mask Description:
      | If input(1) = 1
      |      output = input(2)
      |  else if input(1) = 0
      |      output = 0
      mask Help: On/off switch.
      mask Display: plot(0,0,100,100,[31,31,32,34,34,32,31,31,0],[50,48,47,48,51,53,51,50,50],[100,75,51],[50,50,97]);disp('?')
  Sum : Sum  Inputs=+-
  filter : TransferFcn  Numerator=[1]  Denominator=[1 0.15]
  Dthetar (ALS) : Outport  Port=1  InitialOutput=0
  wires:
  filter/1 -> KHdot/2(input u)
  Sum/1 -> filter/1
  On/Off/1(out) -> Dthetar (ALS)/1
  DHdot r (ALS)/1 -> Sum/1
  ALS?/1 -> On/Off/1(crit)
  KHdot/1(y = K*u) -> On/Off/2(in)
  Hdot-Hdot0/1 -> Sum/2
  V/1 -> KHdot/1(V)

== system apilot3/ap_s/GS ==
  note: Glideslope coupled mode
  GS coupled? : Inport  Port=1  PortWidth=-1  SampleTime=-1
  epsilon_gs : Inport  Port=2  PortWidth=-1  SampleTime=-1
  d(epsilon_gs)/dt : Inport  Port=3  PortWidth=-1  SampleTime=-1
  V : Inport  Port=4  PortWidth=-1  SampleTime=-1
  H : Inport  Port=5  PortWidth=-1  SampleTime=-1
  Keps_gs : Subsystem
      mask Display: plot(0,0,100,100,[0,100,0],[0,50,100]);disp('K(u1)      ')
  Kr : Gain  Gain=1
  On/Off : Subsystem
      mask Type: On/off switch
      mask Description:
      | If input(1) = 1
      |      output = input(2)
      |  else if input(1) = 0
      |      output = 0
      mask Help: On/off switch.
      mask Display: plot(0,0,100,100,[31,31,32,34,34,32,31,31,0],[50,48,47,48,51,53,51,50,50],[100,75,51],[50,50,97]);disp('?')
  Rgs approximation : Fcn  Expr=(u[1]-HRW)/sin(abs(gamgs*pi/180)) + xgs
  Sum : Sum  Inputs=++
  prod : Product  Inputs=2
  Dthetar (GS) : Outport  Port=1  InitialOutput=0
  wires:
  H/1 -> Rgs approximation/1
  GS coupled?/1 -> On/Off/1(crit)
  V/1 -> Keps_gs/1(V)
  epsilon_gs/1 -> Sum/1
  d(epsilon_gs)/dt/1 -> Kr/1
  Kr/1 -> Sum/2
  Sum/1 -> prod/1
  Rgs approximation/1 -> prod/2
  prod/1 -> Keps_gs/2(input u)
  Keps_gs/1(y = K*u) -> On/Off/2(in)
  On/Off/1(out) -> Dthetar (GS)/1

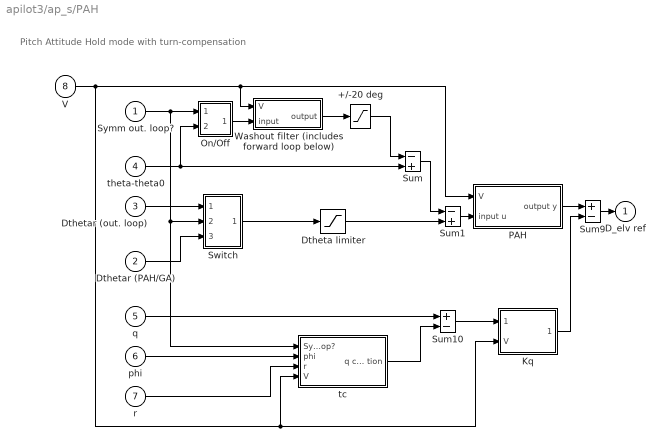
== system apilot3/ap_s/PAH ==
  note: Pitch Attitude Hold mode
      | with turn-compensation
  Symm out. loop? : Inport  Port=1  PortWidth=-1  SampleTime=-1
  Dthetar (PAH/GA) : Inport  Port=2  PortWidth=-1  SampleTime=-1
  Dthetar (out. loop) : Inport  Port=3  PortWidth=-1  SampleTime=-1
  theta-theta0 : Inport  Port=4  PortWidth=-1  SampleTime=-1
  q : Inport  Port=5  PortWidth=-1  SampleTime=-1
  phi : Inport  Port=6  PortWidth=-1  SampleTime=-1
  r : Inport  Port=7  PortWidth=-1  SampleTime=-1
  V : Inport  Port=8  PortWidth=-1  SampleTime=-1
  +/-20 deg : Saturate  UpperLimit=20*(pi/180)  LowerLimit=-20*(pi/180)
  Dtheta limiter : Saturate  UpperLimit=18*(pi/180)  LowerLimit=-8*(pi/180)
  Kq : Subsystem
      mask Display: plot(0,0,100,100,[0,100,0],[0,50,100]);disp('K(u2)      ')
  On/Off : Subsystem
      mask Type: On/off switch
      mask Description:
      | If input(1) = 1
      |      output = input(2)
      |  else if input(1) = 0
      |      output = 0
      mask Help: On/off switch. \nIf input(1) = 1, the output equals input(2). \nIf input(1) = 0, the output is zero.
      mask Display: plot(0,0,100,100,[31,31,32,34,34,32,31,31,0],[50,48,47,48,51,53,51,50,50],[100,75,51],[50,50,97]);disp('?')
  PAH : Subsystem
      mask Display: disp('PAH (limited \n PI controller)')
  Sum : Sum  Inputs=-+
  Sum1 : Sum  Inputs=-+
  Sum10 : Sum  Inputs=+-
  Sum9 : Sum  Inputs=+-
  Switch : Subsystem
      mask Display: plot(0,0,100,100,[100,70,40,0],[50,50,80,80],[40,0],[20,20],[29,29,0],[64,50,50],[29,29],[36,50],[40,40,41,40,39,40],[80,82,80,78,80,82],[40,40,41,40,39,40],[19,21,20,18,20,23])
  Washout filter (includes forward loop below) : Subsystem
      mask Display: disp('Kd/(s+Kd)')
  tc : Subsystem
      mask Display: disp('Turn\nCompensator')
  D_elv ref : Outport  Port=1  InitialOutput=0
  wires:
  Dthetar (PAH/GA)/1 -> Switch/3(Dthetar (PAH/RAH))
  theta-theta0/1 -> On/Off/2(in), Sum/2
  +/-20 deg/1 -> Sum/1
  Sum/1 -> Sum1/1
  tc/1(q correc- tion) -> Sum10/2
  V/1 -> Washout filter (includes forward loop below)/1(V), PAH/1(V), tc/4(V), Kq/2(V)
  Kq/1(y = K*u) -> Sum9/2
  q/1 -> Sum10/1
  Sum10/1 -> Kq/1(input u)
  PAH/1(output y) -> Sum9/1
  Dtheta limiter/1 -> Sum1/2
  Sum1/1 -> PAH/2(input u)
  Sum9/1 -> D_elv ref/1
  On/Off/1(out) -> Washout filter (includes forward loop below)/2(input)
  Washout filter (includes forward loop below)/1(output) -> +/-20 deg/1
  phi/1 -> tc/2(phi)
  r/1 -> tc/3(r)
  Switch/1(Dthetar) -> Dtheta limiter/1
  Dthetar (out. loop)/1 -> Switch/1(Dthetar (out. loop))
  Symm out. loop?/1 -> Switch/2(Symm.  out. loop?), tc/1(Symm. outer loop?), On/Off/1(crit.)

== system apilot3/ap_s/Symm. mode On/Off ==
  crit : Inport  Port=1  PortWidth=-1  SampleTime=-1
  in : Inport  Port=2  PortWidth=-1  SampleTime=-1
  Sum : Sum  Inputs=+-
  Switch : Switch  Threshold=0
  const. : Constant  Value=0.5
  const.1 : Constant  Value=0
  out : Outport  Port=1  InitialOutput=0
  wires:
  const./1 -> Sum/2
  in/1 -> Switch/1
  Switch/1 -> out/1
  Sum/1 -> Switch/2
  const.1/1 -> Switch/3
  crit/1 -> Sum/1

== system apilot3/ap_s/s_cvar ==
  note: Deviations from nominal
      | outputs from AC model:
  note: True values of output
      | signals from AC model:
  note: SELECT SYMM CONTROL VARIABLES.
  z-z0 : Inport  Port=1  PortWidth=-1  SampleTime=-1
  z : Inport  Port=2  PortWidth=-1  SampleTime=-1
  Demux : Demux  Outputs=[7 1 3 1 1]
  Demux1 : Demux  Outputs=[1 3 1 1 2 1 2 1 1]
  Terminator_{1..6} (6 alike) : Terminator
  Hdot-Hdot0 : Outport  Port=1  InitialOutput=0
  H-H0 : Outport  Port=2  InitialOutput=0
  theta-theta0 : Outport  Port=3  InitialOutput=0
  q : Outport  Port=4  InitialOutput=0
  phi : Outport  Port=5  InitialOutput=0
  r : Outport  Port=6  InitialOutput=0
  V : Outport  Port=7  InitialOutput=0
  H : Outport  Port=8  InitialOutput=0
  wires:
  Demux/2 -> theta-theta0/1
  Demux/4 -> H-H0/1
  Demux/5 -> Hdot-Hdot0/1
  Demux/3 -> Terminator_2/1
  Demux/1 -> Terminator_1/1
  z-z0/1 -> Demux/1
  Demux1/8 -> H/1
  Demux1/6 -> phi/1
  Demux1/4 -> r/1
  Demux1/3 -> q/1
  Demux1/1 -> V/1
  Demux1/9 -> Terminator_6/1
  Demux1/7 -> Terminator_5/1
  Demux1/5 -> Terminator_4/1
  Demux1/2 -> Terminator_3/1
  z/1 -> Demux1/1

== system apilot3/ap_s/s_mc ==
  note: SELECT SYMM REFERENCE SIGNALS
  note: SELECT SYMM MODE (on/off flags denoted by '?')
  ymode : Inport  Port=1  PortWidth=-1  SampleTime=-1
  yref : Inport  Port=2  PortWidth=-1  SampleTime=-1
  Demux : Demux  Outputs=[1 1 1 1 1 5]
  Demux1 : Demux  Outputs=[1 1 1 2]
  Terminator_1 : Terminator
  Terminator_2 : Terminator
  symm mode? : Outport  Port=1  InitialOutput=0
  symm. outer loop? : Outport  Port=2  InitialOutput=0
  Dthetar (PAH) : Outport  Port=3  InitialOutput=0
  ALS? : Outport  Port=4  InitialOutput=0
  DHdot r (ALS) : Outport  Port=5  InitialOutput=0
  ALH? : Outport  Port=6  InitialOutput=0
  DHr (ALH) : Outport  Port=7  InitialOutput=0
  GS coupled? : Outport  Port=8  InitialOutput=0
  wires:
  Demux/6 -> Terminator_1/1
  ymode/1 -> Demux/1
  Demux1/4 -> Terminator_2/1
  yref/1 -> Demux1/1
  Demux/2 -> symm. outer loop?/1
  Demux/1 -> symm mode?/1
  Demux/3 -> ALH?/1
  Demux/4 -> ALS?/1
  Demux/5 -> GS coupled?/1
  Demux1/1 -> Dthetar (PAH)/1
  Demux1/2 -> DHr (ALH)/1
  Demux1/3 -> DHdot r (ALS)/1

== system apilot3/ap_s/t ==

== system apilot3/d+l/t ==

== system apilot3/sens/H ==
  H in : Inport  Port=1  PortWidth=-1  SampleTime=-1
  1 = cont. signal 2 = 4ft quantizer 3 = MA-filter : Constant  Value=1
  3-switch : Subsystem
      mask Display: disp('Switch:\ny=u(u[1]+1)')
  4ft quantizer : Fcn  Expr=u-rem(u,q)  mask(Quantizer){@1=4*0.3048}
      mask prompts: @1 "Quantization interval:"
      mask help: Discretizes input at given interval.
      mask init:
      | q = @1;
      mask Help: Quantizes input in given intervals.
      mask Display: plot([10,0],[5,5],[5,5],[0,10],[1,2,2,3,3,4,4,5,5,6,6,7,7,8,8,9,9],[1,1,2,2,3,3,4,4,5,5,6,6,7,7,8,8,9])
  MA-filter : DiscreteStateSpace  A=Ama  B=Bma  C=Cma  D=Dma  X0=xinit  SampleTime=Ts  mask(MA-filter){@1=10, @2=0.033, @3=0}
      mask prompts: @1 "Number of samples for averaging:"; @2 "Sample time:"; @3 "Initial value of input signal:"
      mask help: Digital Moving Average filter
      mask init:
      | ns=@1; Ama=[zeros(1,ns);[eye(ns-1) zeros(ns-1,1)]]; Bma=[1; zeros(ns-1,1)]; Cma=1/ns*ones(1,ns); Dma=0; Ts=@2; uinit=@3; xinit=uinit*ones(ns,1);
      mask Help: Digital Moving Average filter. \ny(k) = 1/n * (u(k) + u(k-1) + ... + u(k-ns)) \nwhere ns is the number of samples \nfor averaging (to be specified by \nthe user).
      mask Display: disp('MA')
  Transport delay static pressure : TransportDelay  DelayTime=0.4  InitialInput=0  BufferSize=1024
  H out : Outport  Port=1  InitialOutput=0
  wires:
  4ft quantizer/1 -> MA-filter/1, 3-switch/3(u2)
  MA-filter/1 -> 3-switch/4(u3)
  1 = cont. signal 2 = 4ft quantizer 3 = MA-filter/1 -> 3-switch/1(Which input?)
  3-switch/1(y) -> H out/1
  H in/1 -> Transport delay static pressure/1
  Transport delay static pressure/1 -> 3-switch/2(u1), 4ft quantizer/1

== system apilot3/sens/Hdot ==
  Hdot in : Inport  Port=1  PortWidth=-1  SampleTime=-1
  Pressure delay/ computing time airdata computer : TransportDelay  DelayTime=0.8  InitialInput=0  BufferSize=1024
  Hdot out : Outport  Port=1  InitialOutput=0
  wires:
  Hdot in/1 -> Pressure delay/ computing time airdata computer/1
  Pressure delay/ computing time airdata computer/1 -> Hdot out/1

== system apilot3/sens/V ==
  V in : Inport  Port=1  PortWidth=-1  SampleTime=-1
  Transport Delay pitot system : TransportDelay  DelayTime=0.4  InitialInput=0  BufferSize=1024
  V out : Outport  Port=1  InitialOutput=0
  wires:
  V in/1 -> Transport Delay pitot system/1
  Transport Delay pitot system/1 -> V out/1

== system apilot3/sens/alpha ==
  alpha in : Inport  Port=1  PortWidth=-1  SampleTime=-1
  alpha out : Outport  Port=1  InitialOutput=0
  wires:
  alpha in/1 -> alpha out/1

== system apilot3/sens/beta ==
  beta in : Inport  Port=1  PortWidth=-1  SampleTime=-1
  beta out : Outport  Port=1  InitialOutput=0
  wires:
  beta in/1 -> beta out/1

== system apilot3/sens/p ==
  p in : Inport  Port=1  PortWidth=-1  SampleTime=-1
  p out : Outport  Port=1  InitialOutput=0
  wires:
  p in/1 -> p out/1

== system apilot3/sens/phi ==
  phi in : Inport  Port=1  PortWidth=-1  SampleTime=-1
  phi out : Outport  Port=1  InitialOutput=0
  wires:
  phi in/1 -> phi out/1

== system apilot3/sens/psi ==
  psi in : Inport  Port=1  PortWidth=-1  SampleTime=-1
  psi out : Outport  Port=1  InitialOutput=0
  wires:
  psi in/1 -> psi out/1

== system apilot3/sens/q ==
  q in : Inport  Port=1  PortWidth=-1  SampleTime=-1
  q out : Outport  Port=1  InitialOutput=0
  wires:
  q in/1 -> q out/1

== system apilot3/sens/r ==
  r in : Inport  Port=1  PortWidth=-1  SampleTime=-1
  r out : Outport  Port=1  InitialOutput=0
  wires:
  r in/1 -> r out/1

== system apilot3/sens/t ==

== system apilot3/sens/theta ==
  theta in : Inport  Port=1  PortWidth=-1  SampleTime=-1
  theta out : Outport  Port=1  InitialOutput=0
  wires:
  theta in/1 -> theta out/1

== system apilot3/w+t/t ==
